simulink model "kiem_chung_xe_day_r2021b"  (R2021b)
settings: Solver=VariableStepAuto  StartTime=0.0  StopTime=1.5  RelTol=1e-3
undefined symbols (not defined in the file): G1, G2, Kdx, Kix, Kpx
settings Model: SimulationMode=accelerator  Creator=datng  LastModifiedBy=datng
settings DebuggingCC: UnconnectedInputMsg=none  UnconnectedOutputMsg=none  UnconnectedLineMsg=none
settings ModelReferenceCC: EnableRefExpFcnMdlSchedulingChecks=off
settings RTWCC: GPUComputeCapability=5.0  DLArmComputeVersion=20.02.1
settings ConfigComp: CovBoundaryAbsTol=1.0e-5

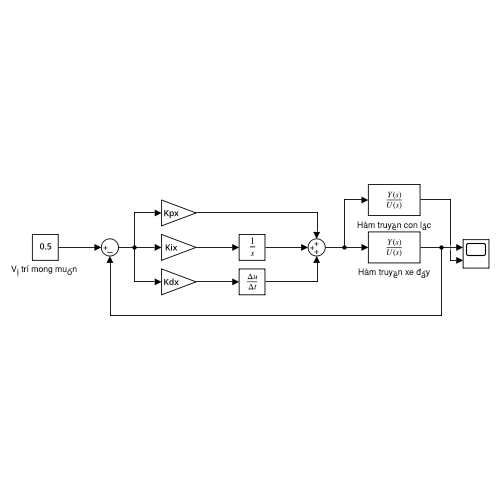
[thumbnail: Simulink's stored preview of the top-level diagram]
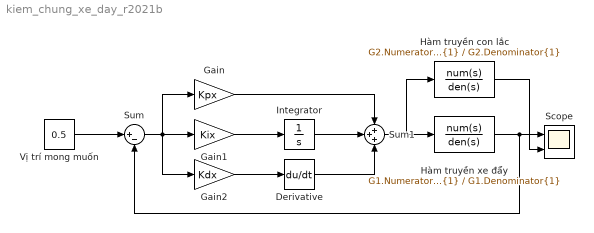
== system kiem_chung_xe_day_r2021b ==
  Derivative : Derivative  CoefficientInTFapproximation=0
  Gain : Gain  Gain=Kpx
  Gain1 : Gain  Gain=Kix
  Gain2 : Gain  Gain=Kdx
  Hàm truyền con lắc : TransferFcn  Numerator=G2.Numerator{1}  Denominator=G2.Denominator{1}
  Hàm truyền xe đẩy : TransferFcn  Numerator=G1.Numerator{1}  Denominator=G1.Denominator{1}
  Integrator : Integrator
  Scope : Scope  NumInputPorts=2
  Sum : Sum  Inputs=|+-
  Sum1 : Sum  Inputs=+++
  "Vị trí mong muốn " : Constant  Value=0.5
  wires:
  "Vị trí mong muốn "/1 -> Sum/1
  Sum/1 -> Gain/1, Gain2/1, Gain1/1
  Gain1/1 -> Integrator/1
  Integrator/1 -> Sum1/2
  Derivative/1 -> Sum1/3
  Gain2/1 -> Derivative/1
  Gain/1 -> Sum1/1
  Sum1/1 -> Hàm truyền con lắc/1, Hàm truyền xe đẩy/1
  Hàm truyền xe đẩy/1 -> Scope/1, Sum/2
  Hàm truyền con lắc/1 -> Scope/2
